simulink model "Boat_model_joystick_simplified"  (Simulink 6.6)
settings: Solver=ode3  StartTime=0.0  StopTime=10000  FixedStep=1  RelTol=1e-3
values from neighbouring files (symbols this model uses):
  C_d_sea_surge = 340    [boat_constants.m]
  d_prop = .4572    (= 0.4572)    [boat_constants.m]
  damping_rudder = 0.01    [boat_constants.m]
  e_0 = 0    [boat_constants.m]
  I_rudder = 0.01    [boat_constants.m]
  K_d_rudder = 200    [boat_constants.m]
  K_i_rudder = 0    [boat_constants.m]
  K_p_rudder = 1000    [boat_constants.m]
  K_t = 0.5    [boat_constants.m]
  mass = 550    [boat_constants.m]
  n_0 = 0    [boat_constants.m]
  phi_0 = 0    [boat_constants.m]
  rho_w = 1.03e3    (= 1030)    [boat_constants.m]
  stiffness_rudder = 0    [boat_constants.m]
  wheelbase = 3.27    [boat_constants.m]
undefined symbols (not defined in the file or in its folder): render_boat
libraries: simulink x2, vrlib x1
settings Model: Creator=Administrator  LastModifiedBy=Administrator

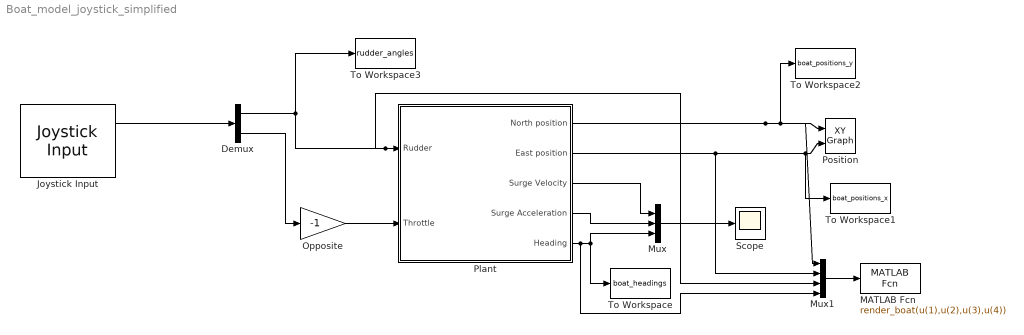
== system Boat_model_joystick_simplified ==
  Demux : Demux  Outputs=3
  Joystick Input : vrlib/Joystick Input  joyid=1  adjustports=on  forcefeed=off
  MATLAB Fcn : MATLABFcn  MATLABFcn=render_boat(u(1),u(2),u(3),u(4))  OutputDimensions=0  Output1D=off
  Mux : Mux  Inputs=3
  Mux1 : Mux
  Opposite : Gain  Gain=-1
  Plant : Subsystem
  Position : simulink/Sinks/XY Graph  SystemSampleTime=-1  xmin=-10000  xmax=10000  ymin=-10000  ymax=10000  st=-1
  Scope : Scope
  To Workspace : ToWorkspace  VariableName=boat_headings  SampleTime=-1  SaveFormat=Array
  To Workspace1 : ToWorkspace  VariableName=boat_positions_x  SampleTime=-1  SaveFormat=Array
  To Workspace2 : ToWorkspace  VariableName=boat_positions_y  SampleTime=-1  SaveFormat=Array
  To Workspace3 : ToWorkspace  VariableName=rudder_angles  SampleTime=-1  SaveFormat=Array
  wires:
  Plant/1(North position) -> Position/1, To Workspace2/1, Mux1/1
  Plant/2(East position) -> Position/2, To Workspace1/1, Mux1/2
  Demux/1 -> To Workspace3/1, Plant/1(Rudder), Mux1/3
  Demux/3 -> Opposite/1
  Joystick Input/1 -> Demux/1
  Plant/3(Surge Velocity) -> Mux/1
  Plant/5(Heading) -> Mux/3, To Workspace/1, Mux1/4
  Plant/4(Surge Acceleration) -> Mux/2
  Mux/1 -> Scope/1
  Mux1/1 -> MATLAB Fcn/1
  Opposite/1 -> Plant/2(Throttle)

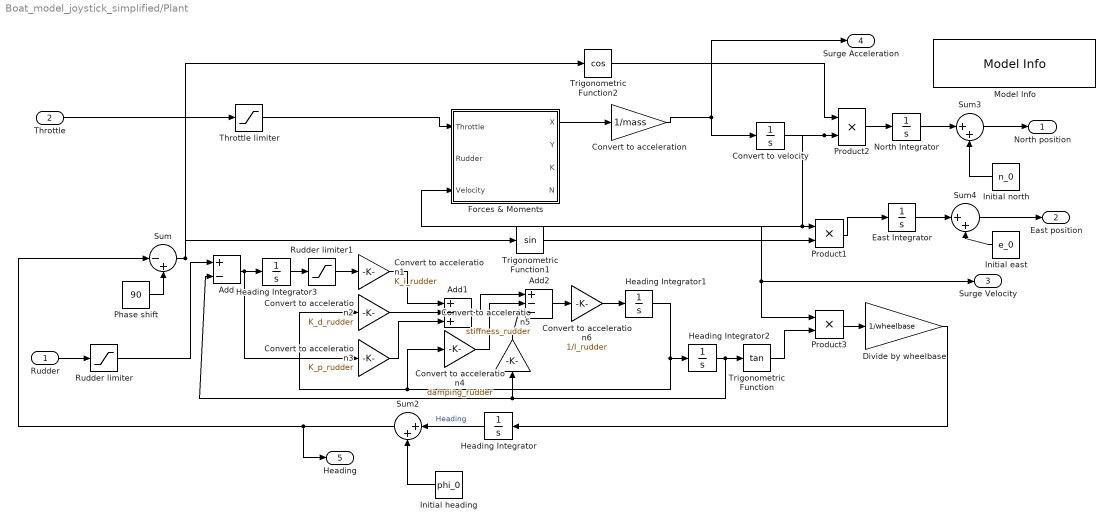
== system Boat_model_joystick_simplified/Plant ==
  Rudder : Inport
  Throttle : Inport  Port=2
  Add : Sum  Inputs=+-  OutScaling=2^-10
  Add1 : Sum  Inputs=+-+  OutScaling=2^-10
  Add2 : Sum  Inputs=+--  OutScaling=2^-10
  Convert to acceleration : Gain  Gain=1/mass
  Convert to acceleration1 : Gain  Gain=K_i_rudder
  Convert to acceleration2 : Gain  Gain=K_d_rudder
  Convert to acceleration3 : Gain  Gain=K_p_rudder
  Convert to acceleration4 : Gain  Gain=damping_rudder
  Convert to acceleration5 : Gain  Orientation=up  Gain=stiffness_rudder
  Convert to acceleration6 : Gain  Gain=1/I_rudder
  Convert to velocity : Integrator
  Divide by wheelbase : Gain  Gain=1/wheelbase
  East Integrator : Integrator
  Forces & Moments : Subsystem
  Heading Integrator : Integrator  Orientation=left
  Heading Integrator1 : Integrator
  Heading Integrator2 : Integrator
  Heading Integrator3 : Integrator
  Initial east : Constant  Orientation=left  Value=e_0
  Initial heading : Constant  Orientation=left  Value=phi_0
  Initial north : Constant  Orientation=left  Value=n_0
  Model Info : simulink/Model-Wide Utilities/Model Info  SystemSampleTime=-1  InitialBlockCM=None  BlockCM=None  Frame=on  DisplayStringWithTags=|  HorizontalTextAlignment=Center  LeftAlignmentValue=0.5  SourceBlockDiagram=Boat_model_joystick_simplified  TagMaxNumber=20
      | Kinematic model of the autoboat.
      | Version %<ModelVersion>
  North Integrator : Integrator
  Phase shift : Constant  Value=90
  Product1 : Product  RndMeth=Zero
  Product2 : Product  RndMeth=Zero
  Product3 : Product  RndMeth=Zero
  Rudder limiter : Saturate  UpperLimit=1  LowerLimit=-1
  Rudder limiter1 : Saturate  UpperLimit=10  LowerLimit=-10
  Sum : Sum  Inputs=|-+
  Sum2 : Sum  Orientation=left  Inputs=|++
  Sum3 : Sum  Inputs=|++
  Sum4 : Sum  Inputs=|++
  Throttle limiter : Saturate  UpperLimit=1  LowerLimit=0
  Trigonometric Function : Trigonometry  Operator=tan  OutputSignalType=real
  Trigonometric Function1 : Trigonometry  OutputSignalType=real
  Trigonometric Function2 : Trigonometry  Operator=cos  OutputSignalType=real
  North position : Outport
  East position : Outport  Port=2
  Surge Velocity : Outport  Port=3
  Surge Acceleration : Outport  Port=4
  Heading : Outport  Port=5
  wires:
  Trigonometric Function2/1 -> Product2/1
  Trigonometric Function1/1 -> Product1/2
  Product2/1 -> North Integrator/1
  Trigonometric Function/1 -> Product3/2
  Product3/1 -> Divide by wheelbase/1
  Sum/1 -> Trigonometric Function2/1, Trigonometric Function1/1
  Product1/1 -> East Integrator/1
  Divide by wheelbase/1 -> Heading Integrator/1
  Convert to velocity/1 -> Product2/2, Product1/1, Product3/1, Forces & Moments/3(Velocity), Surge Velocity/1
  Convert to acceleration/1 -> Convert to velocity/1, Surge Acceleration/1
  Forces & Moments/1(X) -> Convert to acceleration/1
  Throttle/1 -> Throttle limiter/1
  Rudder/1 -> Rudder limiter/1
  Phase shift/1 -> Sum/2
  Heading Integrator/1 -> Sum2/1  "Heading"
  Initial heading/1 -> Sum2/2
  Sum2/1 -> Heading/1, Sum/1
  Initial north/1 -> Sum3/2
  North Integrator/1 -> Sum3/1
  Sum3/1 -> North position/1
  East Integrator/1 -> Sum4/1
  Sum4/1 -> East position/1
  Initial east/1 -> Sum4/2
  Throttle limiter/1 -> Forces & Moments/1(Throttle)
  Rudder limiter/1 -> Add/1
  Add/1 -> Heading Integrator3/1, Convert to acceleration3/1
  Convert to acceleration1/1 -> Add1/1
  Convert to acceleration2/1 -> Add1/2
  Heading Integrator1/1 -> Heading Integrator2/1, Convert to acceleration2/1, Convert to acceleration4/1
  Heading Integrator2/1 -> Trigonometric Function/1, Convert to acceleration5/1, Add/2
  Convert to acceleration3/1 -> Add1/3
  Add1/1 -> Add2/1
  Convert to acceleration4/1 -> Add2/2
  Convert to acceleration5/1 -> Add2/3
  Add2/1 -> Convert to acceleration6/1
  Convert to acceleration6/1 -> Heading Integrator1/1
  Heading Integrator3/1 -> Rudder limiter1/1
  Rudder limiter1/1 -> Convert to acceleration1/1

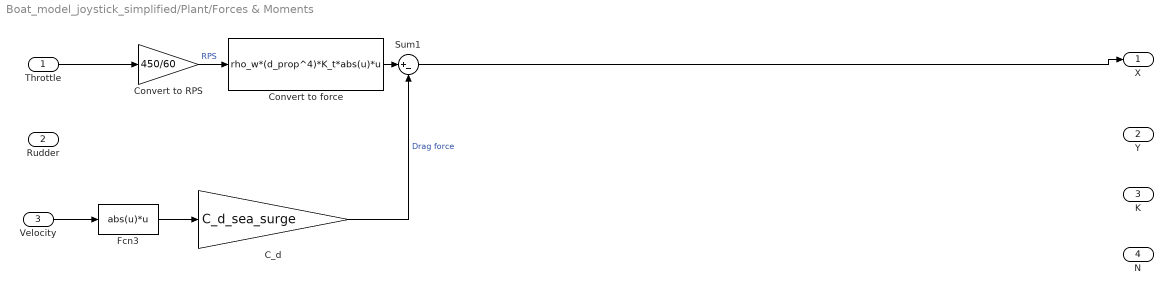
== system Boat_model_joystick_simplified/Plant/Forces & Moments ==
  Throttle : Inport
  Rudder : Inport  Port=2
  Velocity : Inport  Port=3
  C_d : Gain  Gain=C_d_sea_surge
  Convert to RPS : Gain  Gain=450/60
  Convert to force : Fcn  Expr=rho_w*(d_prop^4)*K_t*abs(u)*u
  Fcn3 : Fcn  Expr=abs(u)*u
  Sum1 : Sum  Inputs=|+-
  X : Outport
  Y : Outport  Port=2
  K : Outport  Port=3
  N : Outport  Port=4
  wires:
  Convert to RPS/1 -> Convert to force/1  "RPS"
  Fcn3/1 -> C_d/1
  C_d/1 -> Sum1/2  "Drag force"
  Convert to force/1 -> Sum1/1
  Velocity/1 -> Fcn3/1
  Throttle/1 -> Convert to RPS/1
  Sum1/1 -> X/1
